simulink library "lib_Convection_SimpNatConvHeatX"  (R2015a)
settings: Solver=ode45  StartTime=0.0  StopTime=10.0  RelTol=1e-3
settings Model: Creator=jlkratz  LastModifiedBy=jlkratz

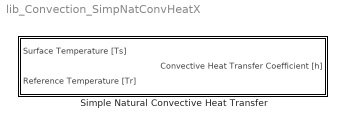
== system lib_Convection_SimpNatConvHeatX ==
  Simple Natural Convective Heat Transfer : Subsystem  mask(Simple Natural Convective Heat Transfer Block (T-SAT)){hcoeff_M=0.03, dTdes_M=1, BN_M=gcb}
      mask prompts: hcoeff_M "hcoeff_M - Convective heat transfer coefficient when W = Wdes and T = Tdes"; dTdes_M "dTdes_M - Design Ts - Tr (known data point)"; BN_M "BN_M - Block name"
      mask help:
      | This block models takes a simplistic apporach at modeling the natural convection heat transfer coefficient (hn). The equation for calculating the convective heat transfer coefficient is based on empirical models and attempts to correlate the heat transfer coefficient with the surface and fluid temperatures (Ts and Tr respectively).
      |
      | h = hcoeff * [(Ts-Tr)/(Ts-Tr)des]^(0.25)
      |
      | In the equation above, Ts-Tr)des is the temperautre difference of the surface and fluid when h = hcoeff. This block can accept various units but the units must be consistent.
      mask Help: web(which('Convection_TSAT_SimpNatConvHeatX.html'),'-helpbrowser')

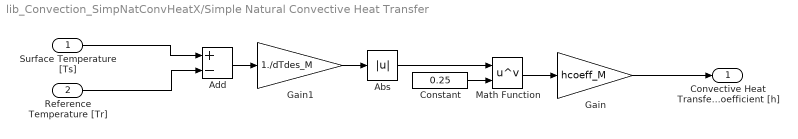
== system lib_Convection_SimpNatConvHeatX/Simple Natural Convective Heat Transfer ==
  "Surface Temperature [Ts] " : Inport
  Reference Temperature [Tr] : Inport  Port=2
  Abs : Abs
  Add : Sum  Inputs=+-
  Constant : Constant  Value=0.25
  Gain : Gain  Gain=hcoeff_M
  Gain1 : Gain  Gain=1./dTdes_M
  Math Function : Math  Operator=pow  SaturateOnIntegerOverflow=on
  Convective Heat Transfer Coefficient [h] : Outport
  wires:
  "Surface Temperature [Ts] "/1 -> Add/1
  Math Function/1 -> Gain/1
  Reference Temperature [Tr]/1 -> Add/2
  Gain/1 -> Convective Heat Transfer Coefficient [h]/1
  Constant/1 -> Math Function/2
  Add/1 -> Gain1/1
  Abs/1 -> Math Function/1
  Gain1/1 -> Abs/1
